simulink library "SUB_ECU_L4_MABX_HW_Interface_PTC_166"  (R2018a)
settings: Solver=VariableStepAuto  StartTime=0.0  StopTime=10.0  RelTol=1e-3
PostLoadFcn:
  | , if any(exist('dsrtsu_mdlpostloadfcn', 'file') == [2, 3, 6]), try dsrtsu_mdlpostloadfcn('Execute', bdroot); catch fprintf('Error in PostLoadFcn (dsrtsu_mdlpostloadfcn) for model "%s":\n %s\n', bdroot, lasterr); end, end,
undefined symbols (not defined in the file or in its folder): CANR_PROPB_REAX_3_13_CHANNEL_APV, CANR_PROPB_REAX_4_13_CHANNEL_APV, CANR_PROPB_XPR_1_50_CHANNEL_APV, ENUM_CAN_RX_T, ENUM_CAN_TX_T, ENUM_REAX_OPERATION_MODE_T, ENUM_SIGNAL_HEALTH_T, ENUM_XBR_CONTROL_MODE_T, ENUM_XBR_EBI_MODE_T, ENUM_XBR_PASS_THROUGH_ACTIVE_T, ENUM_XBR_PRIORITY_T, ENUM_XPR_INHIBIT_PARK_MANUAL_T, ENUM_XPR_INHIBIT_UNPARK_MANUAL_T, ENUM_XPR_PARK_MANUAL_T, ENUM_XPR_UNPARK_MANUAL_T, PROPB_REAX_1_E4_DES_POS_SIG_SRC_APV, PROPB_REAX_1_E4_DESIRED_OPMODE_APV, PROPB_REAX_1_E4_DESIRED_POSITION_APV, ptc_matlab_lib
libraries: PTC_MBDS_LIB x163, rtican x79, simulink x41, EmE_MBD_Blockset x35, rti1401lib_dio_type4 x8, simulink_need_slupdate x7, $bdroot x5, rti1401lib_adc_type4 x3, rtitasklib x1
(part 4 of 25)

== system SUB_ECU_L4_MABX_HW_Interface_PTC_166/CAN_Truck166/CAN_RX_AIR1_31 ==
  Constant : Constant  Value=boolean(1)
  RX_CAN_1 : Subsystem
  AIR1_31 : Outport
  wires:
  RX_CAN_1/1(AIR1_31) -> AIR1_31/1
  Constant/1 -> RX_CAN_1/1(Enable)

== system SUB_ECU_L4_MABX_HW_Interface_PTC_166/CAN_Truck166/CAN_RX_AMB_00 ==
  Constant : Constant  Value=boolean(1)
  RX_CAN_1 : Subsystem
  AMB_00 : Outport
  wires:
  Constant/1 -> RX_CAN_1/1(Enable)
  RX_CAN_1/1(AMB_00) -> AMB_00/1

== system SUB_ECU_L4_MABX_HW_Interface_PTC_166/CAN_Truck166/CAN_RX_B2_31 ==
  Constant : Constant
  RX_CAN_4 : Subsystem
  B2_00 : Outport
  wires:
  RX_CAN_4/1(B2_31) -> B2_00/1
  Constant/1 -> RX_CAN_4/1(Enable)

== system SUB_ECU_L4_MABX_HW_Interface_PTC_166/CAN_Truck166/CAN_RX_Bendix_RADAR_Tracks ==
  Constant : Constant  Value=boolean(1)
  RX_CAN_1 : Subsystem
  Bendix_RADAR_Tracks : Outport
  wires:
  RX_CAN_1/1(Bendix_RADAR_Tracks) -> Bendix_RADAR_Tracks/1
  Constant/1 -> RX_CAN_1/1(Enable)

== system SUB_ECU_L4_MABX_HW_Interface_PTC_166/CAN_Truck166/CAN_RX_CCVS1_00 ==
  Constant : Constant  Value=boolean(1)
  RX_CAN_1 : Subsystem
  CCVS1_0 : Outport
  wires:
  Constant/1 -> RX_CAN_1/1(Enable)
  RX_CAN_1/1(CCVS1_0) -> CCVS1_0/1

== system SUB_ECU_L4_MABX_HW_Interface_PTC_166/CAN_Truck166/CAN_RX_CCVS1_31 ==
  Constant : Constant  Value=boolean(1)
  RX_CAN_31 : Subsystem
  CCVS1_31 : Outport
  wires:
  RX_CAN_31/1(CCVS1_31_) -> CCVS1_31/1
  Constant/1 -> RX_CAN_31/1(Enable)

== system SUB_ECU_L4_MABX_HW_Interface_PTC_166/CAN_Truck166/CAN_RX_COGSOGRapidUpdate_01 ==
  Constant : Constant
  RX_CAN_4 : Subsystem
  COGSOGRapidUpdate_01 : Outport
  wires:
  Constant/1 -> RX_CAN_4/1(Enable)
  RX_CAN_4/1(COGSOGRapidUpdate_01) -> COGSOGRapidUpdate_01/1

== system SUB_ECU_L4_MABX_HW_Interface_PTC_166/CAN_Truck166/CAN_RX_CVW_0B ==
  Constant : Constant  Value=boolean(1)
  RX_CAN_1 : Subsystem
  CVW_0B : Outport
  wires:
  Constant/1 -> RX_CAN_1/1(Enable)
  RX_CAN_1/1(CVW_0B) -> CVW_0B/1

== system SUB_ECU_L4_MABX_HW_Interface_PTC_166/CAN_Truck166/CAN_RX_EBC1_0B ==
  Constant1 : Constant  Value=boolean(1)
  RX_CAN_1_EBC1 : Subsystem
  EBC1_0B : Outport
  wires:
  Constant1/1 -> RX_CAN_1_EBC1/1(Enable)
  RX_CAN_1_EBC1/1(EBC1_0B_) -> EBC1_0B/1

== system SUB_ECU_L4_MABX_HW_Interface_PTC_166/CAN_Truck166/CAN_RX_EBC1_8B ==
  Constant1 : Constant  Value=boolean(1)
  RX_CAN_5_EBC1 : Subsystem
  EBC1_8B : Outport
  wires:
  RX_CAN_5_EBC1/1(EBC1_8B) -> EBC1_8B/1
  Constant1/1 -> RX_CAN_5_EBC1/1(Enable)

== system SUB_ECU_L4_MABX_HW_Interface_PTC_166/CAN_Truck166/CAN_RX_EBC2_0B ==
  Enable_RX_EBC2_0B : Constant  Value=boolean(1)
  RX_CAN_1 : Subsystem
  EBC2_0B : Outport
  wires:
  Enable_RX_EBC2_0B/1 -> RX_CAN_1/1(Enable)
  RX_CAN_1/1(EBC2_0B) -> EBC2_0B/1

== system SUB_ECU_L4_MABX_HW_Interface_PTC_166/CAN_Truck166/CAN_RX_EC1_00 ==
  TPCM_BAM_CAN1 : Inport
  TPDT_BAM_CAN1 : Inport  Port=2
  timeStamp : Inport  Port=3
  Bus Creator : BusCreator  Inputs=5
  Bus Selector13 : BusSelector  OutputSignals=RX_status
  Bus Selector5 : BusSelector  OutputSignals=Signals.TPCM_BAM.SPN2569_ParameterGroupNumber
  CAN_RX_EC1_00 : Subsystem  TreatAsAtomicUnit=on
  Constant2 : Constant  Value=uint32(hex2dec('FEE3'))
  Decode_EC1 : PTC_MBDS_LIB/J1939/Decoders/Decode_EC1  PTC_MBDS_BlockVersion=5.41  PTC_BlockType=PTC_MBDS_Decode_EC1
      settings: SourceProductName=PACCAR Technical Center MBDS Library
  EQ1 : PTC_MBDS_LIB/MBDS Standard Library/Basic Operations/Logic and Bit Operations/EQ  InputSameDT=on  PTC_MBDS_BlockVersion=5.41  PTC_BlockType=PTC_MBDS_EQ
      settings: SourceProductName=PACCAR Technical Center MBDS Library
  Logical Operator : Logic  AllPortsSameDT=off  OutDataTypeStr=boolean
  EC1_00 : Outport
  wires:
  timeStamp/1 -> CAN_RX_EC1_00/3(timeStamp)
  Logical Operator/1 -> CAN_RX_EC1_00/Enable
  Decode_EC1/1 -> [Signals]
  CAN_RX_EC1_00/2(RX_status) -> [RX_status]
  CAN_RX_EC1_00/4(RX_delta_time) -> [RX_delta_time]
  CAN_RX_EC1_00/3(RX_time) -> [RX_time]
  CAN_RX_EC1_00/1(RawData) -> Decode_EC1/1, [RawData]
  Bus Creator/1 -> EC1_00/1
  TPDT_BAM_CAN1/1 -> [TPDT_BAM_CAN1]
  [RX_delta_time] -> Bus Creator/5
  [RawData] -> Bus Creator/2
  [RX_status] -> Bus Creator/3
  [Signals] -> Bus Creator/1
  [RX_time] -> Bus Creator/4
  [TPDT_BAM_CAN1] -> CAN_RX_EC1_00/2(TPDT)
  [TPCM_BAM_CAN1] -> CAN_RX_EC1_00/1(TPCM)
  TPCM_BAM_CAN1/1 -> [TPCM_BAM_CAN1]
  Constant2/1 -> EQ1/2
  EQ1/1 -> Logical Operator/2
  [TPCM_BAM_CAN1] -> Bus Selector5/1
  Bus Selector5/1 -> EQ1/1  "<SPN2569_ParameterGroupNumber>"
  [TPDT_BAM_CAN1] -> Bus Selector13/1
  Bus Selector13/1 -> Logical Operator/1  "<RX_status>"

== system SUB_ECU_L4_MABX_HW_Interface_PTC_166/CAN_Truck166/CAN_RX_EEC1_00 ==
  Enable_RX_EEC1_00 : Constant  Value=boolean(1)
  RX_CAN_1 : Subsystem
  EEC1_00 : Outport
  wires:
  Enable_RX_EEC1_00/1 -> RX_CAN_1/1(Enable)
  RX_CAN_1/1(EEC1_00) -> EEC1_00/1

== system SUB_ECU_L4_MABX_HW_Interface_PTC_166/CAN_Truck166/CAN_RX_EEC2_00 ==
  Enable_RX_EEC2_00 : Constant  Value=boolean(1)
  RX_CAN_2 : Subsystem
  EEC2_00 : Outport
  wires:
  RX_CAN_2/1(EEC2_00) -> EEC2_00/1
  Enable_RX_EEC2_00/1 -> RX_CAN_2/1(Enable)

== system SUB_ECU_L4_MABX_HW_Interface_PTC_166/CAN_Truck166/CAN_RX_EEC3_00 ==
  Enable_RX_EEC3_00 : Constant  Value=boolean(1)
  RX_CAN_1 : Subsystem
  EEC3_00 : Outport
  wires:
  Enable_RX_EEC3_00/1 -> RX_CAN_1/1(Enable)
  RX_CAN_1/1(EEC3_00) -> EEC3_00/1

== system SUB_ECU_L4_MABX_HW_Interface_PTC_166/CAN_Truck166/CAN_RX_ETC2_03 ==
  Enable_RX_ETC2_03 : Constant  Value=boolean(1)
  RX_CAN_1 : Subsystem
  ETC2_03 : Outport
  wires:
  Enable_RX_ETC2_03/1 -> RX_CAN_1/1(Enable)
  RX_CAN_1/1(ETC2_03) -> ETC2_03/1

== system SUB_ECU_L4_MABX_HW_Interface_PTC_166/CAN_Truck166/CAN_RX_GNSSDOPs_00 ==
  Constant : Constant
  RX_CAN_4 : Subsystem
  GNSSDOPs_00 : Outport
  wires:
  Constant/1 -> RX_CAN_4/1(Enable)
  RX_CAN_4/1(GNSSDOPs_00) -> GNSSDOPs_00/1

== system SUB_ECU_L4_MABX_HW_Interface_PTC_166/CAN_Truck166/CAN_RX_HRW_0B ==
  Enable_HRW_RX_0B : Constant  Value=boolean(1)
  RX_CAN_1 : Subsystem
  HRW_0B : Outport
  wires:
  RX_CAN_1/1(HRW_0B_) -> HRW_0B/1
  Enable_HRW_RX_0B/1 -> RX_CAN_1/1(Enable)

== system SUB_ECU_L4_MABX_HW_Interface_PTC_166/CAN_Truck166/CAN_RX_PROPB_REAX_2_13 ==
  In1 : Inport
  Bus Selector : BusSelector  OutputSignals=EnablePropB_ReAX_CAN5,EnablePropB_ReAX_CAN4
  RX_CAN_4 : Subsystem
  RX_CAN_5 : Subsystem
  Switch : Switch  Criteria=u2 ~= 0
  PROPB_REAX_2_13 : Outport
  wires:
  Switch/1 -> PROPB_REAX_2_13/1
  RX_CAN_4/1(PROPB_REAX_2_13) -> Switch/3
  Bus Selector/2 -> RX_CAN_4/1(Enable)  "<EnablePropB_ReAX_CAN4>"
  Bus Selector/1 -> RX_CAN_5/1(Enable), Switch/2  "<EnablePropB_ReAX_CAN5>"
  In1/1 -> Bus Selector/1
  RX_CAN_5/1(PROPB_REAX_2_13) -> Switch/1

== system SUB_ECU_L4_MABX_HW_Interface_PTC_166/CAN_Truck166/CAN_RX_PROPB_REAX_3_13 ==
  Constant : Constant  Value=CANR_PROPB_REAX_3_13_CHANNEL_APV
  Multiport_Switch : MultiPortSwitch  DataPortOrder=Specify indices  DataPortIndices={ENUM_CAN_RX_T.RX_CAN_1, ENUM_CAN_RX_T.RX_CAN_2, ENUM_CAN_RX_T.RX_CAN_3, ENUM_CAN_RX_T.RX_CAN_4, ENUM_CAN_RX_T.RX_CAN_5, ENUM_CAN_RX_T.RX_CAN_6}  DataPortForDefault=Additional data port  SaturateOnIntegerOverflow=on  InputSameDT=on
      settings: AttributesFormatString=Zero-based indexing: %<zeroidx>
  RX_CAN_1 : Subsystem
  SelectChannel : Subsystem
  Terminator{,1..4} (5 alike) : Terminator
      settings: InitFcn=|
      | try
      |    MBDS_BlockCallback('Update', gcb);
      | end
  PROPB_REAX_3_13 : Outport
  wires:
  RX_CAN_1/1(PROPB_REAX_3_13) -> Multiport_Switch/2, Multiport_Switch/8, Multiport_Switch/7, Multiport_Switch/6, Multiport_Switch/5, Multiport_Switch/4, Multiport_Switch/3
  Constant/1 -> SelectChannel/1(In1), Multiport_Switch/1
  SelectChannel/1(CAN1) -> RX_CAN_1/1(Enable)
  SelectChannel/6(CAN6) -> Terminator4/1
  SelectChannel/5(CAN5) -> Terminator3/1
  SelectChannel/4(CAN4) -> Terminator2/1
  SelectChannel/3(CAN3) -> Terminator1/1
  SelectChannel/2(CAN2) -> Terminator/1
  Multiport_Switch/1 -> PROPB_REAX_3_13/1

== system SUB_ECU_L4_MABX_HW_Interface_PTC_166/CAN_Truck166/CAN_RX_PROPB_REAX_4_13 ==
  Constant : Constant  Value=CANR_PROPB_REAX_4_13_CHANNEL_APV
  Multiport_Switch : MultiPortSwitch  DataPortOrder=Specify indices  DataPortIndices={ENUM_CAN_RX_T.RX_CAN_1, ENUM_CAN_RX_T.RX_CAN_2, ENUM_CAN_RX_T.RX_CAN_3, ENUM_CAN_RX_T.RX_CAN_4, ENUM_CAN_RX_T.RX_CAN_5, ENUM_CAN_RX_T.RX_CAN_6}  DataPortForDefault=Additional data port  SaturateOnIntegerOverflow=on  InputSameDT=on
      settings: AttributesFormatString=Zero-based indexing: %<zeroidx>
  RX_CAN_1 : Subsystem
  SelectChannel : Subsystem
  Terminator{,1..4} (5 alike) : Terminator
      settings: InitFcn=|
      | try
      |    MBDS_BlockCallback('Update', gcb);
      | end
  PROPB_REAX_4_13 : Outport
  wires:
  RX_CAN_1/1(PROPB_REAX_4_13) -> Multiport_Switch/2, Multiport_Switch/8, Multiport_Switch/7, Multiport_Switch/6, Multiport_Switch/5, Multiport_Switch/4, Multiport_Switch/3
  Multiport_Switch/1 -> PROPB_REAX_4_13/1
  SelectChannel/2(CAN2) -> Terminator/1
  SelectChannel/3(CAN3) -> Terminator1/1
  SelectChannel/4(CAN4) -> Terminator2/1
  SelectChannel/5(CAN5) -> Terminator3/1
  SelectChannel/6(CAN6) -> Terminator4/1
  SelectChannel/1(CAN1) -> RX_CAN_1/1(Enable)
  Constant/1 -> Multiport_Switch/1, SelectChannel/1(In1)

== system SUB_ECU_L4_MABX_HW_Interface_PTC_166/CAN_Truck166/CAN_RX_PROPB_XPR_1_50 ==
  Constant : Constant  Value=CANR_PROPB_XPR_1_50_CHANNEL_APV
  Multiport_Switch : MultiPortSwitch  DataPortOrder=Specify indices  DataPortIndices={ENUM_CAN_RX_T.RX_CAN_1, ENUM_CAN_RX_T.RX_CAN_2, ENUM_CAN_RX_T.RX_CAN_3, ENUM_CAN_RX_T.RX_CAN_4, ENUM_CAN_RX_T.RX_CAN_5, ENUM_CAN_RX_T.RX_CAN_6}  DataPortForDefault=Additional data port  SaturateOnIntegerOverflow=on  InputSameDT=on
      settings: AttributesFormatString=Zero-based indexing: %<zeroidx>
  RX_CAN_1 : Subsystem
  SelectChannel : Subsystem
  Terminator{,1..4} (5 alike) : Terminator
      settings: InitFcn=|
      | try
      |    MBDS_BlockCallback('Update', gcb);
      | end
  PROPB_XPR_1 : Outport
  wires:
  RX_CAN_1/1(PROPB_XPR_1_50) -> Multiport_Switch/2, Multiport_Switch/8, Multiport_Switch/7, Multiport_Switch/6, Multiport_Switch/5, Multiport_Switch/4, Multiport_Switch/3
  Multiport_Switch/1 -> PROPB_XPR_1/1
  SelectChannel/2(CAN2) -> Terminator/1
  SelectChannel/3(CAN3) -> Terminator1/1
  SelectChannel/4(CAN4) -> Terminator2/1
  SelectChannel/5(CAN5) -> Terminator3/1
  SelectChannel/6(CAN6) -> Terminator4/1
  SelectChannel/1(CAN1) -> RX_CAN_1/1(Enable)
  Constant/1 -> Multiport_Switch/1, SelectChannel/1(In1)

== system SUB_ECU_L4_MABX_HW_Interface_PTC_166/CAN_Truck166/CAN_RX_PX2 ==
  Constant : Constant  Value=boolean(1)
  RX_CAN_6 : Subsystem
  PX2_Lane : Outport
  wires:
  RX_CAN_6/1(PX2_Lane_) -> PX2_Lane/1
  Constant/1 -> RX_CAN_6/1(Enable)

== system SUB_ECU_L4_MABX_HW_Interface_PTC_166/CAN_Truck166/CAN_RX_PosRapidUpdate_01 ==
  In1 : Inport
  Constant : Constant
  RX_CAN_4 : Subsystem
  PosRapidUpdate_01 : Outport
  wires:
  In1/1 -> RX_CAN_4/2(In)
  Constant/1 -> RX_CAN_4/1(Enable)
  RX_CAN_4/1(PosRapidUpdate_01) -> PosRapidUpdate_01/1

== system SUB_ECU_L4_MABX_HW_Interface_PTC_166/CAN_Truck166/CAN_RX_Prop2C2_Status_30 ==
  Constant : Constant
  RX_CAN_1 : Subsystem
  Prop2C2_Status_30 : Outport
  wires:
  RX_CAN_1/1(Prop2C2_Status_30) -> Prop2C2_Status_30/1
  Constant/1 -> RX_CAN_1/1(Enable)

== system SUB_ECU_L4_MABX_HW_Interface_PTC_166/CAN_Truck166/CAN_RX_SSI2_03 ==
  Constant : Constant
  RX_CAN_1 : Subsystem
  SSI2_03 : Outport
  wires:
  Constant/1 -> RX_CAN_1/1(Enable)
  RX_CAN_1/1(SSI2_03) -> SSI2_03/1

== system SUB_ECU_L4_MABX_HW_Interface_PTC_166/CAN_Truck166/CAN_RX_STD_PROPB_PX2_1_E2 ==
  CAN_RX-Enable_PX2_MapLaneEgoLeft : Constant  Value=boolean(1)
  RX_CAN_6 : Subsystem
  PX2_MapLaneEgoLeft : Outport
  wires:
  CAN_RX-Enable_PX2_MapLaneEgoLeft/1 -> RX_CAN_6/1(Enable)
  RX_CAN_6/1(CAN_RX_PX2_MapLaneEgoLeft) -> PX2_MapLaneEgoLeft/1

== system SUB_ECU_L4_MABX_HW_Interface_PTC_166/CAN_Truck166/CAN_RX_STD_PROPB_PX2_1_E3 ==
  CAN_RX-Enable_PX2_MapLaneEgoLeft : Constant  Value=boolean(1)
  RX_CAN_6 : Subsystem
  PX2_MapLaneEgoRight : Outport
  wires:
  RX_CAN_6/1(CAN_RX_PX2_MapLaneEgoRight) -> PX2_MapLaneEgoRight/1
  CAN_RX-Enable_PX2_MapLaneEgoLeft/1 -> RX_CAN_6/1(Enable)

== system SUB_ECU_L4_MABX_HW_Interface_PTC_166/CAN_Truck166/CAN_RX_STD_PROPB_PX2_1_E5 ==
  Constant : Constant  Value=boolean(1)
  RX_CAN_6 : Subsystem
  STD_PROPB_PX2_1_E5 : Outport
  wires:
  Constant/1 -> RX_CAN_6/1(Enable)
  RX_CAN_6/1(STD_PROPB_PX2_1_E5) -> STD_PROPB_PX2_1_E5/1

== system SUB_ECU_L4_MABX_HW_Interface_PTC_166/CAN_Truck166/CAN_RX_SystemTime_01 ==
  Constant : Constant
  RX_CAN_4 : Subsystem
  SystemTime_00 : Outport
  wires:
  Constant/1 -> RX_CAN_4/1(Enable)
  RX_CAN_4/1(SystemTime_00) -> SystemTime_00/1

== system SUB_ECU_L4_MABX_HW_Interface_PTC_166/CAN_Truck166/CAN_RX_TC1_05 ==
  Constant : Constant  Value=boolean(1)
  RX_CAN_5 : Subsystem
  TC1_05 : Outport
  wires:
  RX_CAN_5/1(TC1_05) -> TC1_05/1
  Constant/1 -> RX_CAN_5/1(Enable)

== system SUB_ECU_L4_MABX_HW_Interface_PTC_166/CAN_Truck166/CAN_RX_VDC1_0B ==
  Constant : Constant  Value=boolean(1)
  RX_CAN_1 : Subsystem
  VDC1_0B : Outport
  wires:
  RX_CAN_1/1(VDC1_0B) -> VDC1_0B/1
  Constant/1 -> RX_CAN_1/1(Enable)

== system SUB_ECU_L4_MABX_HW_Interface_PTC_166/CAN_Truck166/CAN_RX_VDC2_0B ==
  Constant : Constant  Value=boolean(1)
  RX_CAN_1 : Subsystem
  VDC2_0B : Outport
  wires:
  Constant/1 -> RX_CAN_1/1(Enable)
  RX_CAN_1/1(VDC2_0B) -> VDC2_0B/1

== system SUB_ECU_L4_MABX_HW_Interface_PTC_166/CAN_Truck166/CAN_RX_VEP1_03 ==
  Constant : Constant
  RX_CAN_1 : Subsystem
  VEP1_03 : Outport
  wires:
  RX_CAN_1/1(VEP1_03) -> VEP1_03/1
  Constant/1 -> RX_CAN_1/1(Enable)

== system SUB_ECU_L4_MABX_HW_Interface_PTC_166/CAN_Truck166/CAN_RX_VI_00 ==
  TPCM_BAM_CAN1 : Inport
  TPDT_BAM_CAN1 : Inport  Port=2
  timeStamp : Inport  Port=3
  Bus Creator : BusCreator  Inputs=5
  Bus Selector13 : BusSelector  OutputSignals=RX_status
  Bus Selector5 : BusSelector  OutputSignals=Signals.TPCM_BAM.SPN2569_ParameterGroupNumber
  CAN_RX_VI_00 : Subsystem  TreatAsAtomicUnit=on
  Constant2 : Constant  Value=uint32(hex2dec('FEEC'))
  Decode_VI : Subsystem
  EQ1 : PTC_MBDS_LIB/MBDS Standard Library/Basic Operations/Logic and Bit Operations/EQ  InputSameDT=on  PTC_MBDS_BlockVersion=5.41  PTC_BlockType=PTC_MBDS_EQ
      settings: SourceProductName=PACCAR Technical Center MBDS Library
  Logical Operator : Logic  AllPortsSameDT=off  OutDataTypeStr=boolean
  VI_00 : Outport
  wires:
  Bus Selector13/1 -> Logical Operator/1  "<RX_status>"
  [TPDT_BAM_CAN1] -> Bus Selector13/1
  Bus Selector5/1 -> EQ1/1  "<SPN2569_ParameterGroupNumber>"
  [TPCM_BAM_CAN1] -> Bus Selector5/1
  EQ1/1 -> Logical Operator/2
  Constant2/1 -> EQ1/2
  TPCM_BAM_CAN1/1 -> [TPCM_BAM_CAN1]
  [TPCM_BAM_CAN1] -> CAN_RX_VI_00/1(TPCM)
  [TPDT_BAM_CAN1] -> CAN_RX_VI_00/2(TPDT)
  [RX_time] -> Bus Creator/4
  [Signals] -> Bus Creator/1
  [RX_status] -> Bus Creator/3
  [RawData] -> Bus Creator/2
  [RX_delta_time] -> Bus Creator/5
  TPDT_BAM_CAN1/1 -> [TPDT_BAM_CAN1]
  Bus Creator/1 -> VI_00/1
  CAN_RX_VI_00/1(RawData) -> [RawData], Decode_VI/1(RawData)
  CAN_RX_VI_00/3(RX_time) -> [RX_time]
  CAN_RX_VI_00/4(RX_delta_time) -> [RX_delta_time]
  CAN_RX_VI_00/2(RX_status) -> [RX_status]
  Decode_VI/1(VI) -> [Signals]
  Logical Operator/1 -> CAN_RX_VI_00/Enable
  timeStamp/1 -> CAN_RX_VI_00/3(timeStamp)

== system SUB_ECU_L4_MABX_HW_Interface_PTC_166/CAN_Truck166/CAN_enable ==
  In1 : Inport
  Bus Creator : BusCreator  Inputs=3
  Bus Selector : BusSelector  OutputSignals=VI_00.Signals.F_Truck1571_VIN_Match,VI_00.Signals.F_Truck166_VIN_Match
  If_Then_Else : EmE_MBD_Blockset/Signal Routing/If_Then_Else
      settings: SourceProductName=PACCAR EmE MBD Blockset
  Logical Operator : Logic  Operator=NOT  OutDataTypeStr=boolean
  Terminator : Terminator
  useGPSSA0 : Constant  Value=boolean(0)
  useGPSSA00 : Constant  Value=boolean(1)
  useReAX_CAN_Ch4 : Constant  Value=true
  Out1 : Outport
  wires:
  Logical Operator/1 -> Bus Creator/2  "EnablePropB_ReAX_CAN5"
  useReAX_CAN_Ch4/1 -> Bus Creator/1, Logical Operator/1  "EnablePropB_ReAX_CAN4"
  useGPSSA0/1 -> If_Then_Else/3
  useGPSSA00/1 -> If_Then_Else/2
  Bus Selector/1 -> If_Then_Else/1  "<F_Truck1571_VIN_Match>"
  If_Then_Else/1 -> Bus Creator/3  "useGPS_SA00"
  Bus Selector/2 -> Terminator/1  "<F_Truck166_VIN_Match>"
  In1/1 -> Bus Selector/1
  Bus Creator/1 -> Out1/1

== system SUB_ECU_L4_MABX_HW_Interface_PTC_166/CAN_Truck166/Decode_PropB_REAX_3 ==
  RawData : Inport  OutDataTypeStr=uint8  PortDimensions=8
  Bus Creator : BusCreator  Inputs=8
  Bus Selector : BusSelector  OutputSignals=byte1
  Bus Selector1 : BusSelector  OutputSignals=byte2
  Bus Selector2 : BusSelector  OutputSignals=byte3,byte4
  Bus Selector3 : BusSelector  OutputSignals=byte5,byte6
  Bus Selector4 : BusSelector  OutputSignals=byte7,byte8
  Demux : Demux  Outputs=8
  MergeBuses : PTC_MBDS_LIB/Extras/Signal Routing/MergeBuses  NumberOfBuses=5  NumberOfBusesPrev=5  PTC_MBDS_BlockVersion=5.41  PTC_BlockType=PTC_MBDS_MergeBuses  DummyParameter=zDZnZ1XhDf
      settings: SourceProductName=PACCAR Technical Center MBDS Library
  decode_byte1 : Subsystem
  decode_byte2 : Subsystem
  decode_byte3_byte4 : Subsystem
  decode_byte5_byte6 : Subsystem
  decode_byte7_byte8 : Subsystem
  PROPB_REAX_3 : Outport
  wires:
  Bus Selector4/2 -> decode_byte7_byte8/2(byte8)  "<byte8>"
  Bus Selector4/1 -> decode_byte7_byte8/1(byte7)  "<byte7>"
  Bus Selector3/2 -> decode_byte5_byte6/2(byte6)  "<byte6>"
  Bus Selector3/1 -> decode_byte5_byte6/1(byte5)  "<byte5>"
  Bus Selector2/2 -> decode_byte3_byte4/2(byte4)  "<byte4>"
  Bus Selector2/1 -> decode_byte3_byte4/1(byte3)  "<byte3>"
  Bus Selector1/1 -> decode_byte2/1(byte2)  "<byte2>"
  Bus Selector/1 -> decode_byte1/1(byte1)  "<byte1>"
  [RawData] -> Bus Selector/1, Bus Selector1/1, Bus Selector2/1, Bus Selector3/1, Bus Selector4/1
  decode_byte7_byte8/1(Out) -> MergeBuses/5
  decode_byte5_byte6/1(Out) -> MergeBuses/4
  decode_byte3_byte4/1(Out) -> MergeBuses/3
  decode_byte1/1(Out) -> MergeBuses/1
  decode_byte2/1(Out) -> MergeBuses/2
  MergeBuses/1 -> PROPB_REAX_3/1  "Signals"
  Bus Creator/1 -> [RawData]
  Demux/8 -> Bus Creator/8  "byte8"
  Demux/7 -> Bus Creator/7  "byte7"
  Demux/6 -> Bus Creator/6  "byte6"
  Demux/5 -> Bus Creator/5  "byte5"
  Demux/4 -> Bus Creator/4  "byte4"
  Demux/3 -> Bus Creator/3  "byte3"
  Demux/2 -> Bus Creator/2  "byte2"
  Demux/1 -> Bus Creator/1  "byte1"
  RawData/1 -> Demux/1

== system SUB_ECU_L4_MABX_HW_Interface_PTC_166/CAN_Truck166/Decode_PropB_REAX_4 ==
  RawData : Inport  OutDataTypeStr=uint8  PortDimensions=8
  Bus Creator : BusCreator  Inputs=8
  Bus Selector : BusSelector  OutputSignals=byte1
  Bus Selector1 : BusSelector  OutputSignals=byte2
  Bus Selector2 : BusSelector  OutputSignals=byte3
  Bus Selector3 : BusSelector  OutputSignals=byte5
  Bus Selector4 : BusSelector  OutputSignals=byte6,byte7
  Bus Selector5 : BusSelector  OutputSignals=byte8
  Demux : Demux  Outputs=8
  MergeBuses : PTC_MBDS_LIB/Extras/Signal Routing/MergeBuses  NumberOfBuses=6  NumberOfBusesPrev=6  PTC_MBDS_BlockVersion=5.41  PTC_BlockType=PTC_MBDS_MergeBuses  DummyParameter=u_5quVVSbT
      settings: SourceProductName=PACCAR Technical Center MBDS Library
  decode_byte1 : Subsystem
  decode_byte2 : Subsystem
  decode_byte3 : Subsystem
  decode_byte5 : Subsystem
  decode_byte6_byte7 : Subsystem
  decode_byte8 : Subsystem
  PROPB_REAX_4 : Outport
  wires:
  decode_byte6_byte7/1(Out) -> MergeBuses/5
  decode_byte8/1(Out) -> MergeBuses/6
  decode_byte5/1(Out) -> MergeBuses/4
  decode_byte3/1(Out) -> MergeBuses/3
  decode_byte2/1(Out) -> MergeBuses/2
  decode_byte1/1(Out) -> MergeBuses/1
  Bus Selector5/1 -> decode_byte8/1(byte8)  "<byte8>"
  Bus Selector4/2 -> decode_byte6_byte7/2(byte7)  "<byte7>"
  Bus Selector4/1 -> decode_byte6_byte7/1(byte6)  "<byte6>"
  Bus Selector3/1 -> decode_byte5/1(byte5)  "<byte5>"
  Bus Selector2/1 -> decode_byte3/1(byte3)  "<byte3>"
  Bus Selector1/1 -> decode_byte2/1(byte2)  "<byte2>"
  Bus Selector/1 -> decode_byte1/1(byte1)  "<byte1>"
  RawData/1 -> Demux/1
  Demux/1 -> Bus Creator/1  "byte1"
  Demux/2 -> Bus Creator/2  "byte2"
  Demux/3 -> Bus Creator/3  "byte3"
  Demux/4 -> Bus Creator/4  "byte4"
  Demux/5 -> Bus Creator/5  "byte5"
  Demux/6 -> Bus Creator/6  "byte6"
  Demux/7 -> Bus Creator/7  "byte7"
  Demux/8 -> Bus Creator/8  "byte8"
  Bus Creator/1 -> [RawData]
  MergeBuses/1 -> PROPB_REAX_4/1  "Signals"
  [RawData] -> Bus Selector4/1, Bus Selector5/1, Bus Selector3/1, Bus Selector2/1, Bus Selector1/1, Bus Selector/1

== system SUB_ECU_L4_MABX_HW_Interface_PTC_166/DIGITAL/PWM pedal input management ==
  Pedal_1_pwm_freq_raw_value : Inport
  Pedal_1_pwm_dc_raw_value : Inport  Port=2
  Pedal_2_pwm_freq_raw_value : Inport  Port=3
  Pedal_2_pwm_dc_raw_value : Inport  Port=4
  Arbitrate pedal position output : Subsystem
  Determine common angle : Subsystem
  Diagnose pedal input signals : Subsystem
  Fault arbitration : Subsystem
  PWM signal filtering conversion : Subsystem
  Synchronization check sensor 1 and 2 : Subsystem
  Pedal_pwm_position : Outport
  wires:
  Arbitrate pedal position output/1(Pedal_pwm_position) -> Pedal_pwm_position/1
  [Pedal_synch_data_F_Hard] -> Arbitrate pedal position output/2(Pedal_synch_data_F_Hard)
  [F_Pedal_pwm_sens_total_failure] -> Arbitrate pedal position output/1(F_Pedal_pwm_sens_total_failure)
  Arbitrate pedal position output/2(DEFAULT_VALUE) -> Determine common angle/6(DEFAULT_VALUE), Fault arbitration/3(DEFAULT_VALUE)
  PWM signal filtering conversion/1(Pedal_1_pwm_undefault) -> Synchronization check sensor 1 and 2/2(Pedal_1_pwm_undefault), Fault arbitration/2(Pedal_1_pwm_undefault)
  PWM signal filtering conversion/2(Pedal_2_pwm_undefault) -> Synchronization check sensor 1 and 2/3(Pedal_2_pwm_undefault), Fault arbitration/5(Pedal_2_pwm_undefault)
  Fault arbitration/2(Pedal_2_pwm_angle_arbitrated) -> Determine common angle/5(Pedal_2_pwm_angle_arbitrated)
  Fault arbitration/1(Pedal_1_pwm_angle_arbitrated) -> Determine common angle/4(Pedal_1_pwm_angle_arbitrated)
  Synchronization check sensor 1 and 2/1(F_Pedal_pwm_sync_fault) -> [F_Pedal_pwm_sync_fault]
  Determine common angle/1(Pedal_pwm_angle_common) -> Arbitrate pedal position output/3(Pedal_pwm_angle_common), Synchronization check sensor 1 and 2/1(Pedal_pwm_angle_common)
  Pedal_1_pwm_freq_raw_value/1 -> Diagnose pedal input signals/1(Pedal_1_pwm_freq_raw_value)
  Pedal_1_pwm_dc_raw_value/1 -> PWM signal filtering conversion/1(Pedal _1_pwm_dc_raw_value), Diagnose pedal input signals/2(Pedal_1_pwm_dc_raw_value)
  Pedal_2_pwm_freq_raw_value/1 -> Diagnose pedal input signals/3(Pedal_2_pwm_freq_raw_value)
  Pedal_2_pwm_dc_raw_value/1 -> Diagnose pedal input signals/4(Pedal_2_pwm_dc_raw_value), PWM signal filtering conversion/2(Pedal _2_pwm_dc_raw_value)
  [F_Pedal_pwm_sync_fault] -> Diagnose pedal input signals/5(F_Pedal_pwm_sync_fault)
  Diagnose pedal input signals/2(F_Pedal_pwm_sens_total_failure) -> Determine common angle/2(F_Pedal_pwm_sens_total_failure), [F_Pedal_pwm_sens_total_failure]
  Diagnose pedal input signals/4(Pedal_synch_data.F_Hard) -> [Pedal_synch_data_F_Hard]
  Diagnose pedal input signals/3(Pedal_2_pwm_health_state) -> Determine common angle/3(Pedal_2_pwm_health_state), Fault arbitration/4(Pedal_2_pwm_health_state)
  Diagnose pedal input signals/1(Pedal_1_pwm_health_state) -> Determine common angle/1(Pedal_1_pwm_health_state), Fault arbitration/1(Pedal_1_pwm_health_state)

== system SUB_ECU_L4_MABX_HW_Interface_PTC_166/DIGITAL/RationalityCheck ==
  UndefaultStatus : Inport
  Chart : Stateflow chart  TreatAsAtomicUnit=on
  DiagPassed : Outport
  wires:
  UndefaultStatus/1 -> Chart/1(Input)
  Chart/1(DiagPassed) -> DiagPassed/1

== system SUB_ECU_L4_MABX_HW_Interface_PTC_166/DIGITAL_out/Determine pedal PWM and duty cycle values ==
  APTC_arb_pedal_position : Inport
  In : Inport  Port=2
  1-D Lookup Table2 : Lookup_n-D  NumberOfTableDimensions=1  BreakpointsForDimension1=[0 100]  Table=[10 45]  ExtrapMethod=Clip  UseLastTableValue=on  InputSameDT=on
      settings: AttributesFormatString=|
      | X: %<BreakpointsForDimension1>
      | Y: %<Table>
  1-D Lookup Table3 : Lookup_n-D  NumberOfTableDimensions=1  BreakpointsForDimension1=[0 100]  Table=[20 90]  ExtrapMethod=Clip  UseLastTableValue=on  InputSameDT=on
      settings: AttributesFormatString=|
      | X: %<BreakpointsForDimension1>
      | Y: %<Table>
  APTC_PEDAL_A_PWM_FREQ_HZ_APV : Constant  Value=200
  APTC_PEDAL_B_PWM_FREQ_HZ_APV : Constant  Value=200
  Bus Selector1 : BusSelector  OutputSignals=INPUTS.DIO_Bus.OperatorEnableSwitch
  Bus Selector4 : BusSelector  OutputSignals=INPUTS.DIO_Bus.Pedal_1_pwm_dc_raw_value
  Bus Selector5 : BusSelector  OutputSignals=INPUTS.DIO_Bus.Pedal_2_pwm_dc_raw_value
  Bus Selector6 : BusSelector  OutputSignals=INPUTS.DIO_Bus.Pedal_1_pwm_freq_raw_value
  Bus Selector7 : BusSelector  OutputSignals=INPUTS.DIO_Bus.Pedal_2_pwm_freq_raw_value
  If_Then_Else{1..2,4..5} (4 alike) : EmE_MBD_Blockset/Signal Routing/If_Then_Else
      settings: SourceProductName=PACCAR EmE MBD Blockset
  Logical Operator : Logic  Operator=NOT  OutDataTypeStr=boolean
  APTC_PWM_pedalA_freq_out : Outport
  APTC_PWM_pedalA_DC_out : Outport  Port=2
  APTC_PWM_pedalB_freq_out : Outport  Port=3
  APTC_PWM_pedalB_DC_out : Outport  Port=4
  wires:
  Bus Selector1/1 -> Logical Operator/1  "<OperatorEnableSwitch>"
  APTC_PEDAL_A_PWM_FREQ_HZ_APV/1 -> If_Then_Else4/3
  APTC_PEDAL_B_PWM_FREQ_HZ_APV/1 -> If_Then_Else5/3
  Bus Selector6/1 -> If_Then_Else4/2  "<Pedal_1_pwm_freq_raw_value>"
  Bus Selector4/1 -> If_Then_Else1/2  "<Pedal_1_pwm_dc_raw_value>"
  Bus Selector7/1 -> If_Then_Else5/2  "<Pedal_2_pwm_freq_raw_value>"
  Logical Operator/1 -> If_Then_Else2/1, If_Then_Else4/1, If_Then_Else5/1, If_Then_Else1/1
  Bus Selector5/1 -> If_Then_Else2/2  "<Pedal_2_pwm_dc_raw_value>"
  1-D Lookup Table3/1 -> If_Then_Else2/3  "PedalPWMB_DC_out"
  1-D Lookup Table2/1 -> If_Then_Else1/3  "PedalPWMA_DC_out"
  In/1 -> Bus Selector1/1, Bus Selector4/1, Bus Selector6/1, Bus Selector7/1, Bus Selector5/1
  APTC_arb_pedal_position/1 -> 1-D Lookup Table2/1, 1-D Lookup Table3/1
  If_Then_Else1/1 -> APTC_PWM_pedalA_DC_out/1
  If_Then_Else2/1 -> APTC_PWM_pedalB_DC_out/1
  If_Then_Else4/1 -> APTC_PWM_pedalA_freq_out/1
  If_Then_Else5/1 -> APTC_PWM_pedalB_freq_out/1

== system SUB_ECU_L4_MABX_HW_Interface_PTC_166/DIGITAL_out/Shift Control ==
  In : Inport
  Bus Creator1 : BusCreator  Inputs=1
  Bus Selector : BusSelector  OutputSignals=INPUTS.DIO_Bus.ShiftControlDC
  Bus Selector1 : BusSelector  OutputSignals=INPUTS.CAN.ETC2_03.SPN524_TransSelectedGear,INPUTS.CAN.ETC2_03.SPN523_TransCurrentGear
  Compare To Zero : simulink/Logic and Bit Operations/Compare To Zero  relop===  OutDataTypeStr=boolean
  Compare To Zero1 : simulink/Logic and Bit Operations/Compare To Zero  relop===  OutDataTypeStr=boolean
  Constant : Constant  Value=.4
  Constant1 : Constant  Value=0.5
  Constant2 : Constant  Value=false
  F_ALLOW_ETC2_FOR_NEUTRAL_OUTPUT_APV : Constant  Value=true
  If_Then_Else : EmE_MBD_Blockset/Signal Routing/If_Then_Else
      settings: SourceProductName=PACCAR EmE MBD Blockset
  Logical Operator : Logic  OutDataTypeStr=boolean
  Logical Operator1 : Logic  OutDataTypeStr=boolean
  Logical Operator2 : Logic  Operator=OR  OutDataTypeStr=boolean
  Relational Operator : RelationalOperator  OutDataTypeStr=boolean  RndMeth=Nearest
  Relational Operator1 : RelationalOperator  Operator=<=  OutDataTypeStr=boolean  RndMeth=Nearest
  Out : Outport
  wires:
  Constant2/1 -> If_Then_Else/3
  F_ALLOW_ETC2_FOR_NEUTRAL_OUTPUT_APV/1 -> If_Then_Else/1
  If_Then_Else/1 -> Logical Operator2/2
  Logical Operator/1 -> Logical Operator2/1
  Logical Operator1/1 -> If_Then_Else/2
  Compare To Zero1/1 -> Logical Operator1/2
  Compare To Zero/1 -> Logical Operator1/1
  Bus Selector1/2 -> Compare To Zero1/1  "<SPN523_TransCurrentGear>"
  Bus Selector1/1 -> Compare To Zero/1  "<SPN524_TransSelectedGear>"
  Bus Selector/1 -> Relational Operator1/1, Relational Operator/1  "<ShiftControlDC>"
  Bus Creator1/1 -> Out/1
  Logical Operator2/1 -> Bus Creator1/1  "Neutral"
  Constant/1 -> Relational Operator/2
  Relational Operator1/1 -> Logical Operator/2
  Relational Operator/1 -> Logical Operator/1
  In/1 -> Bus Selector/1, Bus Selector1/1
  Constant1/1 -> Relational Operator1/2

== system SUB_ECU_L4_MABX_HW_Interface_PTC_166/INPUTS_PTC_166/Timer_Access ==
  IncrementTimer : Subsystem
  Rate Transition : RateTransition  Deterministic=off
  Timer Interrupt : rtitasklib/Timer Interrupt  DSProperties=struct('RTI',struct('Version',uint32(3),'BlockType',struct('isSLSource',uint8(1),'isSLSink',uint8(0),'isHWSource',uint8(0),'isHWSink',uint8(0),'isSetup',uint8(0),'isInline',uint8(1),'isNonInline',uint8(0),'isInterrupt',uint8(1),'isChannelwise',uint8(0)),'IOBoardType','INTLIB','UnitType','TMRINT','Identifier','TMRINT','DialogType','ML','BlockSet','NONE','SlaveProcessor','NONE','RelationId',struct('TH',struct('BlockId','TMRINT'))))  RTIBlockInterface=struct('OutputPortsActive',1,'OutputPortsWidth',int32(1),'FunctionCall',uint32(0),'OutputPortsName',{{[' ']}},'BlockDisplay',{{['DS1401 Board\nTimer B interrupt'],'center'}},'IconTransparency','on','InitLevel',3,'BlockName',struct('Token',{{['Timer Interrupt']}}),'DialogFcn','rtitasklibtmrintgui','SampleTime',{{-1}},'Options',{{'SS_OPTION_FORCE_NONINLINED_FCNCALL','SS_OPTION_ASYNCHRONOUS_INTERRUPT'}})  RTIBlockParameters=struct('ThPeriod',{{'0.01','OFF',[]}},'SampleTime',{{'-1','OFF',[]}},'ThTimerId',{{2,'OFF',[]}},'ThSrcSgnName',{{['Timer B interrupt'],'OFF',[]}},'ThBlk',{{['struct(''blkh'',[''SUB_ECU_L4_MABX_HW_Interface_PTC_166/INPUTS_PTC_166/Timer_Access/Timer Interrupt''],''srcId'',''TIMERB'',''srcSgnId'',''TIMERB'',''intervalTmrBlockId'',[],''srcSgnName'',[''Timer B interrupt''],''srcCpuId'','''',''isSrcCpu'',1,''isTargetCpu'',1,''srcOnMasterCpu'',1,''boardType'','''',''boardTypeNo'','''',''boardNo'',1,''intNo'',0,''subIntNo'',-1,''period'',''0.01'',''entryPoint'',''rti_TIMERB'',''blockName'',[''Timer Interrupt''],''taskNameDisplayExt'','''',''taskType'',''TMRINT'',''groupId'',''B'',''hookFcn'',''NULL'',''isTimerTaskSrc'',0,''service'',''S_PERIODIC_B'',''mpBlkId'','''',''taskPriorityPreConfig'',''none'',''taskPriority'',-1,''taskSortWeighting'',[],''taskSchedulingPolicy'',''FCFS'',''taskOvrPreConfig'',''none'',''taskOvrStrategy'',1,''taskOvrQueueSize'',1,''taskVisibility'',''on'',''taskGroupId'','''',''taskGroupDisplayOrder'',[],''serviceDynamicGen'',0,''disableCodeGen'',0,''boardBase'',''0'',''noBoardBase'','''')'],'OFF',[]}},'TLCFileName',{{'rtitasklibtmrint','OFF',[]}})  RTISFcnParameters=struct('ThBlk','struct','TLCFileName','char','SampleTime','double')  RTIBlockParaDefault=struct('ThPeriod',0.01,'SampleTime',-1,'ThTimerId',2,'ThSrcSgnName',['Timer B interrupt'],'ThBlk',['struct(''srcSgnId'', '''')'],'TLCFileName','rtitasklibtmrint')
  TimeStamp : Outport
  wires:
  Timer Interrupt/1 -> IncrementTimer/Trigger
  IncrementTimer/1(Out1) -> Rate Transition/1
  Rate Transition/1 -> TimeStamp/1  "GLB_Absolute_Timestamp"

== system SUB_ECU_L4_MABX_HW_Interface_PTC_166/CAN_Out_PTC_166/CAN_TX_1000ms/CAN_TX_AIR1_31 ==
  Channel : Inport  OutDataTypeStr=Enum: ENUM_CAN_TX_T
  Data : Inport  Port=2
  AND : PTC_MBDS_LIB/MBDS Standard Library/Basic Operations/Logic and Bit Operations/AND  BitwiseMode=on  Inputs=1  UseBitMask=on  BitMask=bin2dec('00000001')  OutDataTypeStr=Inherit: Inherit via back propagation  PTC_MBDS_BlockVersion=5.41  PTC_BlockType=PTC_MBDS_AND
      settings: AttributesFormatString=bitwise  SourceProductName=PACCAR Technical Center MBDS Library
  AND1 : PTC_MBDS_LIB/MBDS Standard Library/Basic Operations/Logic and Bit Operations/AND  BitwiseMode=on  Inputs=1  UseBitMask=on  BitMask=bin2dec('00000010')  OutDataTypeStr=Inherit: Inherit via back propagation  PTC_MBDS_BlockVersion=5.41  PTC_BlockType=PTC_MBDS_AND
      settings: AttributesFormatString=bitwise  SourceProductName=PACCAR Technical Center MBDS Library
  AND2 : PTC_MBDS_LIB/MBDS Standard Library/Basic Operations/Logic and Bit Operations/AND  BitwiseMode=on  Inputs=1  UseBitMask=on  BitMask=bin2dec('00000100')  OutDataTypeStr=Inherit: Inherit via back propagation  PTC_MBDS_BlockVersion=5.41  PTC_BlockType=PTC_MBDS_AND
      settings: AttributesFormatString=bitwise  SourceProductName=PACCAR Technical Center MBDS Library
  AND3 : PTC_MBDS_LIB/MBDS Standard Library/Basic Operations/Logic and Bit Operations/AND  BitwiseMode=on  Inputs=1  UseBitMask=on  BitMask=bin2dec('00001000')  OutDataTypeStr=Inherit: Inherit via back propagation  PTC_MBDS_BlockVersion=5.41  PTC_BlockType=PTC_MBDS_AND
      settings: AttributesFormatString=bitwise  SourceProductName=PACCAR Technical Center MBDS Library
  AND4 : PTC_MBDS_LIB/MBDS Standard Library/Basic Operations/Logic and Bit Operations/AND  BitwiseMode=on  Inputs=1  UseBitMask=on  BitMask=bin2dec('00010000')  OutDataTypeStr=Inherit: Inherit via back propagation  PTC_MBDS_BlockVersion=5.41  PTC_BlockType=PTC_MBDS_AND
      settings: AttributesFormatString=bitwise  SourceProductName=PACCAR Technical Center MBDS Library
  AND5 : PTC_MBDS_LIB/MBDS Standard Library/Basic Operations/Logic and Bit Operations/AND  BitwiseMode=on  Inputs=1  UseBitMask=on  BitMask=bin2dec('00100000')  OutDataTypeStr=Inherit: Inherit via back propagation  PTC_MBDS_BlockVersion=5.41  PTC_BlockType=PTC_MBDS_AND
      settings: AttributesFormatString=bitwise  SourceProductName=PACCAR Technical Center MBDS Library
  Data Type Conversion : DataTypeConversion  OutDataTypeStr=uint8  SaturateOnIntegerOverflow=on
  Data Type Conversion{2..7} (6 alike) : DataTypeConversion  OutDataTypeStr=boolean  SaturateOnIntegerOverflow=on
  "Shift_Arithmetic " : ArithShift  BitShiftNumber=1
  Shift_Arithmetic 1 : ArithShift  BitShiftNumber=2
  Shift_Arithmetic 2 : ArithShift  BitShiftNumber=3
  Shift_Arithmetic 3 : ArithShift  BitShiftNumber=4
  Shift_Arithmetic 4 : ArithShift  BitShiftNumber=5
  TX_CAN4 : Subsystem
  Terminator{,1..4} (5 alike) : Terminator
  wires:
  Shift_Arithmetic 4/1 -> Data Type Conversion7/1
  AND5/1 -> Shift_Arithmetic 4/1
  Shift_Arithmetic 3/1 -> Data Type Conversion6/1
  AND4/1 -> Shift_Arithmetic 3/1
  Shift_Arithmetic 2/1 -> Data Type Conversion5/1
  AND3/1 -> Shift_Arithmetic 2/1
  Shift_Arithmetic 1/1 -> Data Type Conversion4/1
  "Shift_Arithmetic "/1 -> Data Type Conversion3/1
  AND/1 -> Data Type Conversion2/1
  Data Type Conversion/1 -> AND2/1, AND3/1, AND5/1, AND4/1, AND1/1, AND/1
  Channel/1 -> Data Type Conversion/1
  AND2/1 -> Shift_Arithmetic 1/1
  AND1/1 -> "Shift_Arithmetic "/1
  Data/1 -> TX_CAN4/2(Data)
  Data Type Conversion2/1 -> Terminator/1
  Data Type Conversion3/1 -> Terminator1/1
  Data Type Conversion4/1 -> Terminator2/1
  Data Type Conversion6/1 -> Terminator3/1
  Data Type Conversion7/1 -> Terminator4/1
  Data Type Conversion5/1 -> TX_CAN4/1(Enable)

== system SUB_ECU_L4_MABX_HW_Interface_PTC_166/CAN_Out_PTC_166/CAN_TX_1000ms/CAN_TX_AMB_00 ==
  Channel : Inport  OutDataTypeStr=Enum: ENUM_CAN_TX_T
  Data : Inport  Port=2
  AND : PTC_MBDS_LIB/MBDS Standard Library/Basic Operations/Logic and Bit Operations/AND  BitwiseMode=on  Inputs=1  UseBitMask=on  BitMask=bin2dec('00000001')  OutDataTypeStr=Inherit: Inherit via back propagation  PTC_MBDS_BlockVersion=5.41  PTC_BlockType=PTC_MBDS_AND
      settings: AttributesFormatString=bitwise  SourceProductName=PACCAR Technical Center MBDS Library
  AND1 : PTC_MBDS_LIB/MBDS Standard Library/Basic Operations/Logic and Bit Operations/AND  BitwiseMode=on  Inputs=1  UseBitMask=on  BitMask=bin2dec('00000010')  OutDataTypeStr=Inherit: Inherit via back propagation  PTC_MBDS_BlockVersion=5.41  PTC_BlockType=PTC_MBDS_AND
      settings: AttributesFormatString=bitwise  SourceProductName=PACCAR Technical Center MBDS Library
  AND2 : PTC_MBDS_LIB/MBDS Standard Library/Basic Operations/Logic and Bit Operations/AND  BitwiseMode=on  Inputs=1  UseBitMask=on  BitMask=bin2dec('00000100')  OutDataTypeStr=Inherit: Inherit via back propagation  PTC_MBDS_BlockVersion=5.41  PTC_BlockType=PTC_MBDS_AND
      settings: AttributesFormatString=bitwise  SourceProductName=PACCAR Technical Center MBDS Library
  AND3 : PTC_MBDS_LIB/MBDS Standard Library/Basic Operations/Logic and Bit Operations/AND  BitwiseMode=on  Inputs=1  UseBitMask=on  BitMask=bin2dec('00001000')  OutDataTypeStr=Inherit: Inherit via back propagation  PTC_MBDS_BlockVersion=5.41  PTC_BlockType=PTC_MBDS_AND
      settings: AttributesFormatString=bitwise  SourceProductName=PACCAR Technical Center MBDS Library
  AND4 : PTC_MBDS_LIB/MBDS Standard Library/Basic Operations/Logic and Bit Operations/AND  BitwiseMode=on  Inputs=1  UseBitMask=on  BitMask=bin2dec('00010000')  OutDataTypeStr=Inherit: Inherit via back propagation  PTC_MBDS_BlockVersion=5.41  PTC_BlockType=PTC_MBDS_AND
      settings: AttributesFormatString=bitwise  SourceProductName=PACCAR Technical Center MBDS Library
  AND5 : PTC_MBDS_LIB/MBDS Standard Library/Basic Operations/Logic and Bit Operations/AND  BitwiseMode=on  Inputs=1  UseBitMask=on  BitMask=bin2dec('00100000')  OutDataTypeStr=Inherit: Inherit via back propagation  PTC_MBDS_BlockVersion=5.41  PTC_BlockType=PTC_MBDS_AND
      settings: AttributesFormatString=bitwise  SourceProductName=PACCAR Technical Center MBDS Library
  Data Type Conversion : DataTypeConversion  OutDataTypeStr=uint8  SaturateOnIntegerOverflow=on
  Data Type Conversion{2..7} (6 alike) : DataTypeConversion  OutDataTypeStr=boolean  SaturateOnIntegerOverflow=on
  "Shift_Arithmetic " : ArithShift  BitShiftNumber=1
  Shift_Arithmetic 1 : ArithShift  BitShiftNumber=2
  Shift_Arithmetic 2 : ArithShift  BitShiftNumber=3
  Shift_Arithmetic 3 : ArithShift  BitShiftNumber=4
  Shift_Arithmetic 4 : ArithShift  BitShiftNumber=5
  TX_CAN4 : Subsystem
  Terminator{,1..4} (5 alike) : Terminator
  wires:
  Data Type Conversion5/1 -> TX_CAN4/1(Enable)
  Data Type Conversion7/1 -> Terminator4/1
  Data Type Conversion6/1 -> Terminator3/1
  Data Type Conversion4/1 -> Terminator2/1
  Data Type Conversion3/1 -> Terminator1/1
  Data Type Conversion2/1 -> Terminator/1
  Data/1 -> TX_CAN4/2(Data)
  AND1/1 -> "Shift_Arithmetic "/1
  AND2/1 -> Shift_Arithmetic 1/1
  Channel/1 -> Data Type Conversion/1
  Data Type Conversion/1 -> AND/1, AND1/1, AND4/1, AND5/1, AND3/1, AND2/1
  AND/1 -> Data Type Conversion2/1
  "Shift_Arithmetic "/1 -> Data Type Conversion3/1
  Shift_Arithmetic 1/1 -> Data Type Conversion4/1
  AND3/1 -> Shift_Arithmetic 2/1
  Shift_Arithmetic 2/1 -> Data Type Conversion5/1
  AND4/1 -> Shift_Arithmetic 3/1
  Shift_Arithmetic 3/1 -> Data Type Conversion6/1
  AND5/1 -> Shift_Arithmetic 4/1
  Shift_Arithmetic 4/1 -> Data Type Conversion7/1

== system SUB_ECU_L4_MABX_HW_Interface_PTC_166/CAN_Out_PTC_166/CAN_TX_100ms/CAN_TX_CCVS1_00 ==
  Data : Inport
  Enable_TX_CCVS1_00 : Constant  Value=boolean(1)
  TX_CAN4 : Subsystem
  TX_CAN5 : Subsystem
  wires:
  Enable_TX_CCVS1_00/1 -> TX_CAN4/1(Enable), TX_CAN5/1(Enable)
  Data/1 -> TX_CAN4/2(Data), TX_CAN5/2(Data)

== system SUB_ECU_L4_MABX_HW_Interface_PTC_166/CAN_Out_PTC_166/CAN_TX_100ms/CAN_TX_PROPB_REAX_5_E4 ==
  enable : Inport
  RawData : Inport  Port=2  OutDataTypeStr=uint8
  Data Type Conversion1 : DataTypeConversion  SaturateOnIntegerOverflow=on
  Ground : Ground
  Ground1 : Ground
  TX_CAN4 : Subsystem
  TX_CAN5 : Subsystem
  Terminator : Terminator
  wires:
  Data Type Conversion1/1 -> TX_CAN5/2(RawData), TX_CAN4/2(RawData)
  RawData/1 -> Data Type Conversion1/1
  enable/1 -> Terminator/1
  Ground/1 -> TX_CAN4/1(Enable)  "EnablePropB_ReAX_CAN4"
  Ground1/1 -> TX_CAN5/1(Enable)  "EnablePropB_ReAX_CAN5"

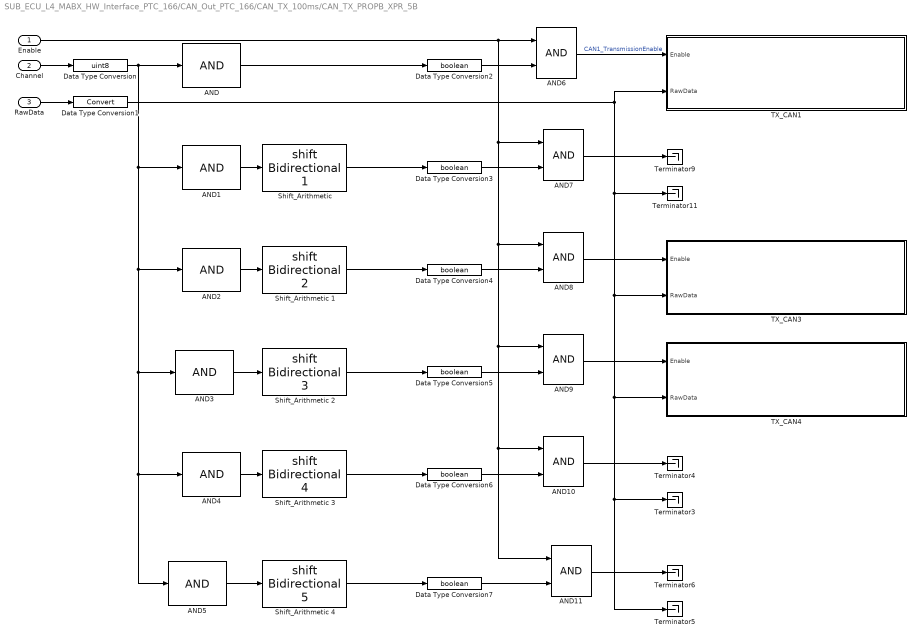
== system SUB_ECU_L4_MABX_HW_Interface_PTC_166/CAN_Out_PTC_166/CAN_TX_100ms/CAN_TX_PROPB_XPR_5B ==
  Enable : Inport
  Channel : Inport  Port=2  OutDataTypeStr=Enum: ENUM_CAN_TX_T
  RawData : Inport  Port=3  OutDataTypeStr=uint8
  AND : PTC_MBDS_LIB/MBDS Standard Library/Basic Operations/Logic and Bit Operations/AND  BitwiseMode=on  Inputs=1  UseBitMask=on  BitMask=bin2dec('00000001')  OutDataTypeStr=Inherit: Inherit via back propagation  PTC_MBDS_BlockVersion=5.41  PTC_BlockType=PTC_MBDS_AND
      settings: AttributesFormatString=bitwise  SourceProductName=PACCAR Technical Center MBDS Library
  AND1 : PTC_MBDS_LIB/MBDS Standard Library/Basic Operations/Logic and Bit Operations/AND  BitwiseMode=on  Inputs=1  UseBitMask=on  BitMask=bin2dec('00000010')  OutDataTypeStr=Inherit: Inherit via back propagation  PTC_MBDS_BlockVersion=5.41  PTC_BlockType=PTC_MBDS_AND
      settings: AttributesFormatString=bitwise  SourceProductName=PACCAR Technical Center MBDS Library
  AND{6..11} (6 alike) : PTC_MBDS_LIB/MBDS Standard Library/Basic Operations/Logic and Bit Operations/AND  BitwiseMode=off  Inputs=2  UseBitMask=off  BitMask='A7'  OutDataTypeStr=Inherit: Inherit via back propagation  PTC_MBDS_BlockVersion=5.41  PTC_BlockType=PTC_MBDS_AND
      settings: SourceProductName=PACCAR Technical Center MBDS Library
  AND2 : PTC_MBDS_LIB/MBDS Standard Library/Basic Operations/Logic and Bit Operations/AND  BitwiseMode=on  Inputs=1  UseBitMask=on  BitMask=bin2dec('00000100')  OutDataTypeStr=Inherit: Inherit via back propagation  PTC_MBDS_BlockVersion=5.41  PTC_BlockType=PTC_MBDS_AND
      settings: AttributesFormatString=bitwise  SourceProductName=PACCAR Technical Center MBDS Library
  AND3 : PTC_MBDS_LIB/MBDS Standard Library/Basic Operations/Logic and Bit Operations/AND  BitwiseMode=on  Inputs=1  UseBitMask=on  BitMask=bin2dec('00001000')  OutDataTypeStr=Inherit: Inherit via back propagation  PTC_MBDS_BlockVersion=5.41  PTC_BlockType=PTC_MBDS_AND
      settings: AttributesFormatString=bitwise  SourceProductName=PACCAR Technical Center MBDS Library
  AND4 : PTC_MBDS_LIB/MBDS Standard Library/Basic Operations/Logic and Bit Operations/AND  BitwiseMode=on  Inputs=1  UseBitMask=on  BitMask=bin2dec('00010000')  OutDataTypeStr=Inherit: Inherit via back propagation  PTC_MBDS_BlockVersion=5.41  PTC_BlockType=PTC_MBDS_AND
      settings: AttributesFormatString=bitwise  SourceProductName=PACCAR Technical Center MBDS Library
  AND5 : PTC_MBDS_LIB/MBDS Standard Library/Basic Operations/Logic and Bit Operations/AND  BitwiseMode=on  Inputs=1  UseBitMask=on  BitMask=bin2dec('00100000')  OutDataTypeStr=Inherit: Inherit via back propagation  PTC_MBDS_BlockVersion=5.41  PTC_BlockType=PTC_MBDS_AND
      settings: AttributesFormatString=bitwise  SourceProductName=PACCAR Technical Center MBDS Library
  Data Type Conversion : DataTypeConversion  OutDataTypeStr=uint8  SaturateOnIntegerOverflow=on
  Data Type Conversion1 : DataTypeConversion  SaturateOnIntegerOverflow=on
  Data Type Conversion{2..7} (6 alike) : DataTypeConversion  OutDataTypeStr=boolean  SaturateOnIntegerOverflow=on
  "Shift_Arithmetic " : ArithShift  BitShiftNumber=1
  Shift_Arithmetic 1 : ArithShift  BitShiftNumber=2
  Shift_Arithmetic 2 : ArithShift  BitShiftNumber=3
  Shift_Arithmetic 3 : ArithShift  BitShiftNumber=4
  Shift_Arithmetic 4 : ArithShift  BitShiftNumber=5
  TX_CAN1 : Subsystem
  TX_CAN3 : Subsystem
  TX_CAN4 : Subsystem
  Terminator{3..6,9,11} (6 alike) : Terminator
  wires:
  AND6/1 -> TX_CAN1/1(Enable)  "CAN1_TransmissionEnable"
  AND7/1 -> Terminator9/1
  AND8/1 -> TX_CAN3/1(Enable)
  AND9/1 -> TX_CAN4/1(Enable)
  AND10/1 -> Terminator4/1
  AND11/1 -> Terminator6/1
  Enable/1 -> AND6/1, AND7/1, AND8/1, AND9/1, AND10/1, AND11/1
  Data Type Conversion7/1 -> AND11/2
  Data Type Conversion6/1 -> AND10/2
  Data Type Conversion5/1 -> AND9/2
  Data Type Conversion4/1 -> AND8/2
  Data Type Conversion3/1 -> AND7/2
  Data Type Conversion2/1 -> AND6/2
  Data Type Conversion1/1 -> Terminator11/1, TX_CAN3/2(RawData), Terminator5/1, Terminator3/1, TX_CAN4/2(RawData), TX_CAN1/2(RawData)
  AND1/1 -> "Shift_Arithmetic "/1
  AND2/1 -> Shift_Arithmetic 1/1
  Channel/1 -> Data Type Conversion/1
  Data Type Conversion/1 -> AND/1, AND1/1, AND4/1, AND5/1, AND3/1, AND2/1
  RawData/1 -> Data Type Conversion1/1
  AND/1 -> Data Type Conversion2/1
  "Shift_Arithmetic "/1 -> Data Type Conversion3/1
  Shift_Arithmetic 1/1 -> Data Type Conversion4/1
  AND3/1 -> Shift_Arithmetic 2/1
  Shift_Arithmetic 2/1 -> Data Type Conversion5/1
  AND4/1 -> Shift_Arithmetic 3/1
  Shift_Arithmetic 3/1 -> Data Type Conversion6/1
  AND5/1 -> Shift_Arithmetic 4/1
  Shift_Arithmetic 4/1 -> Data Type Conversion7/1
